simulink model "rtwdemo_counter"  (Simulink 7.6)
settings: Solver=FixedStepDiscrete  StartTime=0.0  StopTime=48  FixedStep=1  RelTol=1e-3  SampleTimeConstraint=STIndependent
PostLoadFcn:
  | INC=uint8(1);LIMIT=uint8(16);RESET=uint8(0);K=int32(2);
libraries: rtwdemowidgets x1
Description:
  | Algorithm Design
settings Model: Creator=The MathWorks Inc.  ParamWorkspaceSource=ReferencedWorkspace  CovMetricSettings=d  ExtModeTrigMode=oneshot  ExtModeArmWhenConnect=off  ExtModeAutoUpdateStatusClock=off
settings MATStruct: SampleTime=1  Offset=0  Priority=[41.0]
settings DataIOCC: LimitDataPoints=off  SaveFormat=StructureWithTime  SaveOutput=off  SaveTime=off  SignalLoggingName=sigsOut
settings OptimizationCC: InlineParams=on  InlineInvariantSignals=on  StateBitsets=on  DataBitsets=on  UseTempVars=on  EfficientFloat2IntCast=on  EfficientMapNaN2IntZero=off  BufferReusableBoundary=off
settings DebuggingCC: CheckExecutionContextPreStartOutputMsg=on  CheckExecutionContextRuntimeOutputMsg=on  SolverPrmCheckMsg=none  IntegerOverflowMsg=none  StrictBusMsg=ErrorOnBusTreatedAsVector
settings HardwareCC: ProdIntDivRoundTo=Zero  ProdEndianess=LittleEndian  ProdHWDeviceType=Generic->32-bit Embedded Processor  TargetHWDeviceType=Generic->32-bit Embedded Processor
settings ModelReferenceCC: UpdateModelReferenceTargets=IfOutOfDate
settings RTWCC: TLCOptions=-p0 -aWarnNonSaturatedBlocks=0  GenerateReport=on  RTWVerbose=off  ProcessScript=grt_make_rtw_hook  LaunchReport=on
settings CodeAppCC: ForceParamTrailComments=on
settings GRTTargetCC: TargetFcnLib=ansi_tfl_tmw.mat

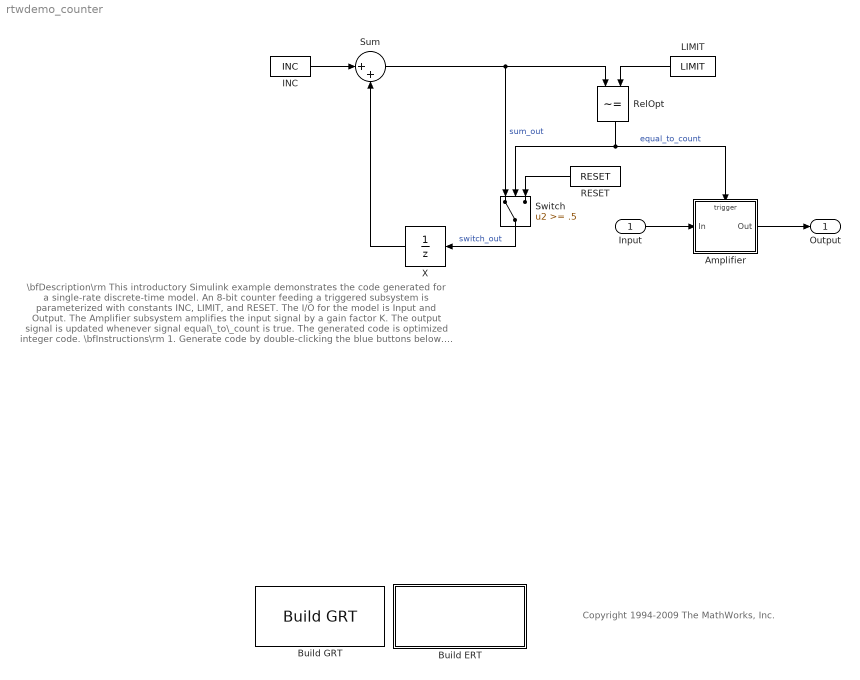
== system rtwdemo_counter ==
  note: \bfDescription\rm
      | This introductory Simulink example demonstrates the code generated for a single-rate
      | discrete-time model.  An 8-bit counter feeding a triggered subsystem is parameterized with
      | constants INC, LIMIT, and RESET.  The I/O for the model is Input and Output. The Amplifier
      | subsystem amplifies the input signal by a gain factor K. The output signal is updated whenever
      | signal equal\_to\_count  is true.  The generated code is optimized integer code.
      |
      | \bfInstructions\rm
      | 1. Generate code by double-clicking the blue buttons below.
      |     An HTML report is displayed automatically.
      | 2. Inspect the generated source files using the hyperlinks embedded in the report.
      |
      | \bfNote\rm
      | Real-Time Workshop uses the GRT code format, which is intended for rapid prototyping.
      | Real-Time Workshop Embedded Coder uses the ERT code format, which is intended for
      | production deployment.
  note: Copyright 1994-2009 The MathWorks, Inc.
  Input : Inport  OutDataTypeStr=int32  PortDimensions=1
  Amplifier : Subsystem  TreatAsAtomicUnit=on
  Build ERT : Subsystem  mask{attrib_overrides={}}
      mask prompts: attrib_overrides "List of attributes to preserve (cell of strings):"
      mask help: Enter the attributes of the configuration set that you want preserved. Otherwise, the default configuration script will override your current settings.
      settings: OpenFcn=|
      | model=bdroot; overrides=get_param(gcb,'attrib_overrides');
      | try
      | 
      | rtwconfiguredemo(model,'noop',false,overrides);
      | 
      | set_param(model,'PurelyIntegerCode','on');
      | set_param(model,'SupportNonFinite','off');
      | set_param(model,'SupportComplex','off');
      | set_param(model,'SupportAbsoluteTime','off');
      | set_param(model,'SupportContinuousTime','off');
      | set_param(model,'SupportNonInlinedSFcns','off');
      | 
      | set_param(model','dirty','off');
      | 
      | rtwbuilddemomodel(model);
      | catch
      |   error(lasterr);
      | end;
      |         clear model overrides;
      mask Display:
      | disp(['Generate Code Using\n',...
      | 	  'Real-Time Workshop\n',...
      | 	  'Embedded Coder\n'...
      | 	  '(double-click)'])
  Build GRT : rtwdemowidgets/Build GRT  SystemSampleTime=-1  attrib_overrides={}
  INC : Constant  Value=INC
  LIMIT : Constant  Value=LIMIT
  RESET : Constant  Value=RESET
  RelOpt : RelationalOperator  Operator=~=  InputSameDT=on
  Sum : Sum  Inputs=|++  InputSameDT=on  OutDataTypeStr=Inherit: Same as first input
  Switch : Switch  Threshold=.5  InputSameDT=on
  X : UnitDelay  SampleTime=-1  StateIdentifier=X
  Output : Outport
  wires:
  INC/1 -> Sum/1
  X/1 -> Sum/2
  Switch/1 -> X/1  "switch_out"
  Sum/1 -> Switch/1, RelOpt/1  "sum_out"
  LIMIT/1 -> RelOpt/2
  Input/1 -> Amplifier/1(In)
  RESET/1 -> Switch/3
  RelOpt/1 -> Switch/2, Amplifier/Trigger  "equal_to_count"
  Amplifier/1(Out) -> Output/1

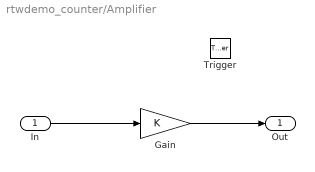
== system rtwdemo_counter/Amplifier ==
  In : Inport
  Trigger : TriggerPort
  Gain : Gain  Gain=K  OutDataTypeStr=Inherit: Same as input  ParamDataTypeStr=Inherit: Same as input
  Out : Outport  InitialOutput=0
  wires:
  In/1 -> Gain/1
  Gain/1 -> Out/1

== system rtwdemo_counter/Build ERT ==
